simulink model "main1"  (Simulink 7.5)
settings: Solver=ode45  StartTime=0.0  StopTime=0.5  RelTol=1e-3
undefined symbols (not defined in the file or in its folder): D1, Delta, DiscIntNeverNeededParam, Hydride, Metal, Nickel
libraries: elec_lib x216, powerlib x83, fl_lib x9, powerlib_extras x8, simulink x3, nesl_utility x2, electricdrivelib x1
(part 1 of 2)
settings Model: Creator=quad  LastModifiedBy=quad

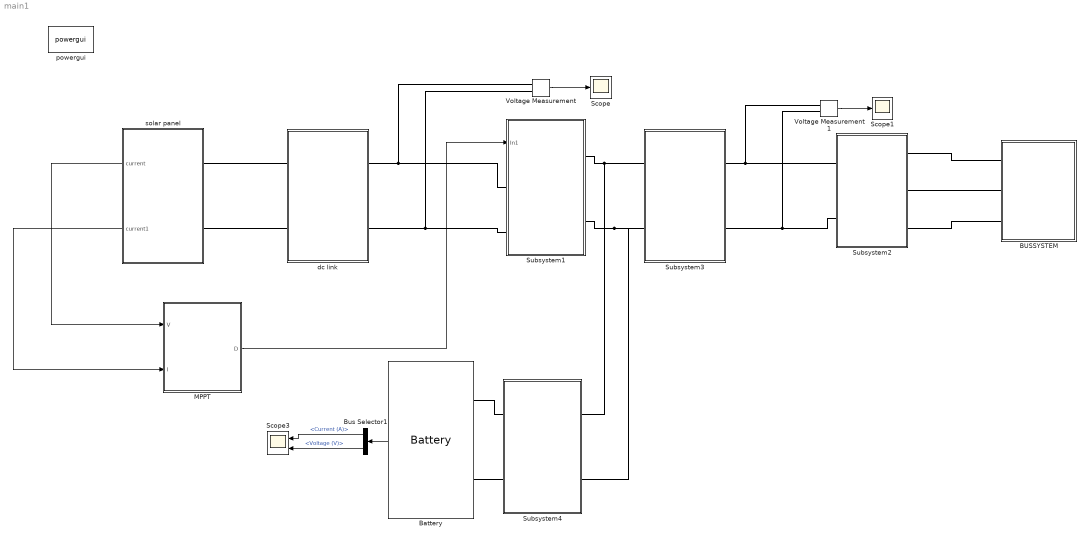
== system main1 ==
  BUSSYSTEM : Subsystem
  Battery : electricdrivelib/Extra Sources/Battery  DialogController=POWERSYS.PowerSysDialog  SystemSampleTime=-1  BatType=Nickel-Metal-Hydride  ShowDetailedParameters=off  NomV=220  NomQ=100  SOC=100  PresetModel=on  MaxQ=107.6923  FullV=259.1525  Dis_rate=20  R=0.022  Normal_OP=96.1538  expZone="[238.6441            20]"  Dis_Char=off  current=[6.5 13 32.5]  Units=Time  Batt_Tr=30
  Bus Selector1 : BusSelector  OutputSignals=Current (A),Voltage (V)
  MPPT : Subsystem
      mask Display: disp('MPPT')
  Scope : Scope
      settings: YMin=75  YMax=115  SaveName=ScopeData6
  Scope1 : Scope
      settings: YMin=0  YMax=1050
  Scope3 : Scope  NumInputPorts=2
      settings: YMin=-0.5~259.4  YMax=9~259.6  SaveName=ScopeData5
  Subsystem1 : Subsystem
      mask Display: disp('Converter')
  Subsystem2 : Subsystem
      mask Display: disp('Inverter')
  Subsystem3 : Subsystem
      mask Display: disp('DC Link')
  Subsystem4 : Subsystem
      mask Display: disp('Converter')
  Voltage Measurement : powerlib/Measurements/Voltage Measurement  DialogController=POWERSYS.PowerSysDialog  SystemSampleTime=-1  PhasorSimulation=off  OutputType=Complex  PSBequivalent=0
  Voltage Measurement1 : powerlib/Measurements/Voltage Measurement  DialogController=POWERSYS.PowerSysDialog  SystemSampleTime=-1  PhasorSimulation=off  OutputType=Complex  PSBequivalent=0
  dc link : Subsystem
      mask Display: disp('DC Link')
  powergui : powerlib/powergui  Priority=1  SystemSampleTime=-1  SimulationMode=Discrete  SampleTime=5e-6  frequency=60  SPID=off  DisableSnubberDevices=off  DisableRonSwitches=off  DisableVfSwitches=off  SwTol=0  Interpol=off  frequencyindice=50  echomessages=off  HookPort=off  DisplayEquations=off  FunctionMessages=off  EnableUseOfTLC=off  x0status=blocks  RestoreLinks=warning  ResistiveCurrentMeasurement=off  Ylog=off  Xlog=on  ShowGrid=off  save=off  variable=ZData  ZoomFFT=off  StartTime=0.0  cycles=1  DisplayStyle=1  FreqAxis=off  MaxFrequency=1000  frequencyindicesteady=1  display=off  methode=off
  solar panel : Subsystem
      mask Display: disp('Solar Panel')
  wires:
  Voltage Measurement/1 -> Scope/1
  Voltage Measurement1/1 -> Scope1/1
  Battery/1 -> Bus Selector1/1
  Bus Selector1/1 -> Scope3/1  "<Current (A)>"
  Bus Selector1/2 -> Scope3/2  "<Voltage (V)>"
  solar panel/1(current) -> MPPT/1(V)
  solar panel/2(current1) -> MPPT/2(I)
  MPPT/1(D) -> Subsystem1/1(In1)
  connections:
  Voltage Measurement/LConn1 -- dc link/RConn1 -- Subsystem1/LConn1
  Voltage Measurement/LConn2 -- dc link/RConn2 -- Subsystem1/LConn2
  Subsystem4/RConn1 -- Subsystem1/RConn1 -- Subsystem3/LConn1
  Subsystem4/RConn2 -- Subsystem1/RConn2 -- Subsystem3/LConn2
  Subsystem2/LConn1 -- Voltage Measurement1/LConn1 -- Subsystem3/RConn1
  Subsystem2/LConn2 -- Voltage Measurement1/LConn2 -- Subsystem3/RConn2
  Battery/LConn2 -- Subsystem4/LConn2
  solar panel/LConn2 -- dc link/LConn2
  solar panel/LConn1 -- dc link/LConn1
  Battery/LConn1 -- Subsystem4/LConn1
  Subsystem2/RConn1 -- BUSSYSTEM/LConn1
  Subsystem2/RConn2 -- BUSSYSTEM/LConn2
  Subsystem2/RConn3 -- BUSSYSTEM/LConn3

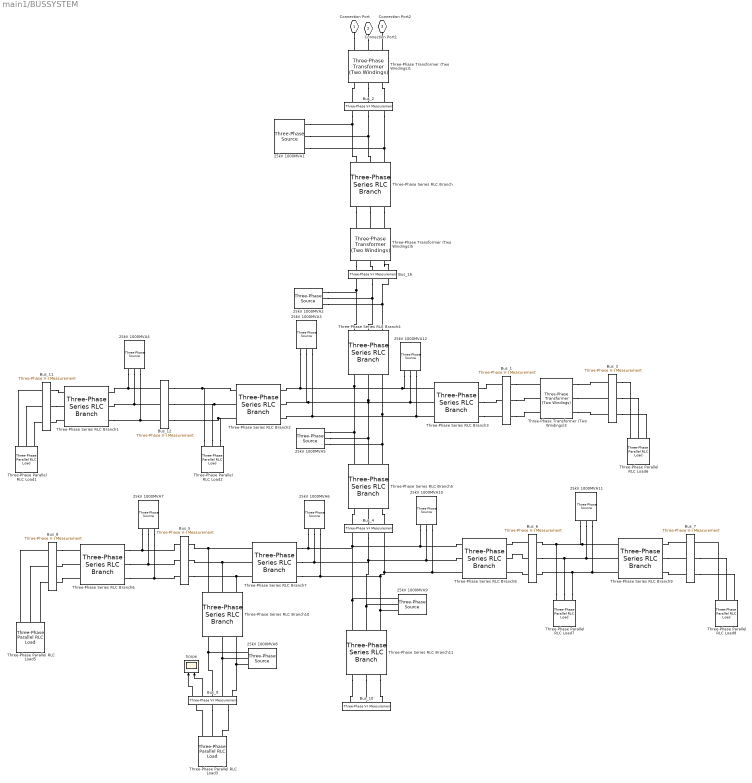
== system main1/BUSSYSTEM ==
  25kV 1000MVA{1..4,6..12} (11 alike) : powerlib/Electrical Sources/Three-Phase Source  DialogController=POWERSYS.PowerSysDialog  SystemSampleTime=-1  Voltage=10  PhaseAngle=0  Frequency=50  InternalConnection=Yg  SpecifyImpedance=on  Resistance=25^2/1000/10  Inductance=25^2/1000/377  ShortCircuitLevel=1000e6  BaseVoltage=25e3  XRratio=10
  25kV 1000MVA5 : powerlib/Electrical Sources/Three-Phase Source  DialogController=POWERSYS.PowerSysDialog  SystemSampleTime=-1  Voltage=25e3  PhaseAngle=0  Frequency=50  InternalConnection=Yg  SpecifyImpedance=on  Resistance=25^2/1000/10  Inductance=25^2/1000/377  ShortCircuitLevel=1000e6  BaseVoltage=25e3  XRratio=10
  Bus_1 : powerlib/Measurements/Three-Phase V-I Measurement  DialogController=POWERSYS.PowerSysDialog  SystemSampleTime=-1  VoltageMeasurement=phase-to-phase  SetLabelV=on  LabelV=Vabc_5  Vpu=off  VpuLL=off  CurrentMeasurement=yes  SetLabelI=on  LabelI=Iabc_5  Ipu=off  Pbase=100e6  Vbase=120e3  OutputType=Complex  PhasorSimulation=on  PSBequivalent=0
      link override Model/VI/Ia: GotoTag=LibraryTag_Ia
      link override Model/VI/Ib: GotoTag=LibraryTag_Ib
      link override Model/VI/Ic: GotoTag=LibraryTag_Ic
      link override Model/VI/Va: GotoTag=LibraryTag_Va
      link override Model/VI/Vb: GotoTag=LibraryTag_Vb
      link override Model/VI/Vc: GotoTag=LibraryTag_Vc
  Bus_10 : powerlib/Measurements/Three-Phase V-I Measurement  DialogController=POWERSYS.PowerSysDialog  SystemSampleTime=-1  VoltageMeasurement=phase-to-phase  SetLabelV=on  LabelV=Vabc_13  Vpu=off  VpuLL=off  CurrentMeasurement=yes  SetLabelI=on  LabelI=Iabc_13  Ipu=off  Pbase=100e6  Vbase=120e3  OutputType=Complex  PhasorSimulation=on  PSBequivalent=0
      link override Model/VI/Ia: GotoTag=LibraryTag_Ia
      link override Model/VI/Ib: GotoTag=LibraryTag_Ib
      link override Model/VI/Ic: GotoTag=LibraryTag_Ic
      link override Model/VI/Va: GotoTag=LibraryTag_Va
      link override Model/VI/Vb: GotoTag=LibraryTag_Vb
      link override Model/VI/Vc: GotoTag=LibraryTag_Vc
  Bus_11 : powerlib/Measurements/Three-Phase V-I Measurement  DialogController=POWERSYS.PowerSysDialog  SystemSampleTime=-1  VoltageMeasurement=phase-to-phase  SetLabelV=on  LabelV=Vabc_3  Vpu=off  VpuLL=off  CurrentMeasurement=yes  SetLabelI=on  LabelI=Iabc_3  Ipu=off  Pbase=100e6  Vbase=120e3  OutputType=Complex  PhasorSimulation=on  PSBequivalent=0
      link override Model/VI/Ia: GotoTag=LibraryTag_Ia
      link override Model/VI/Ib: GotoTag=LibraryTag_Ib
      link override Model/VI/Ic: GotoTag=LibraryTag_Ic
      link override Model/VI/Va: GotoTag=LibraryTag_Va
      link override Model/VI/Vb: GotoTag=LibraryTag_Vb
      link override Model/VI/Vc: GotoTag=LibraryTag_Vc
  Bus_12 : powerlib/Measurements/Three-Phase V-I Measurement  DialogController=POWERSYS.PowerSysDialog  SystemSampleTime=-1  VoltageMeasurement=phase-to-phase  SetLabelV=on  LabelV=Vabc_4  Vpu=off  VpuLL=off  CurrentMeasurement=yes  SetLabelI=on  LabelI=Iabc_4  Ipu=off  Pbase=100e6  Vbase=120e3  OutputType=Complex  PhasorSimulation=on  PSBequivalent=0
      link override Model/VI/Ia: GotoTag=LibraryTag_Ia
      link override Model/VI/Ib: GotoTag=LibraryTag_Ib
      link override Model/VI/Ic: GotoTag=LibraryTag_Ic
      link override Model/VI/Va: GotoTag=LibraryTag_Va
      link override Model/VI/Vb: GotoTag=LibraryTag_Vb
      link override Model/VI/Vc: GotoTag=LibraryTag_Vc
  Bus_16 : powerlib/Measurements/Three-Phase V-I Measurement  DialogController=POWERSYS.PowerSysDialog  SystemSampleTime=-1  VoltageMeasurement=phase-to-phase  SetLabelV=on  LabelV=Vabc_1  Vpu=off  VpuLL=off  CurrentMeasurement=yes  SetLabelI=on  LabelI=Iabc_1  Ipu=off  Pbase=100e6  Vbase=120e3  OutputType=Complex  PhasorSimulation=on  PSBequivalent=0
      link override Model/VI/Ia: GotoTag=LibraryTag_Ia
      link override Model/VI/Ib: GotoTag=LibraryTag_Ib
      link override Model/VI/Ic: GotoTag=LibraryTag_Ic
      link override Model/VI/Va: GotoTag=LibraryTag_Va
      link override Model/VI/Vb: GotoTag=LibraryTag_Vb
      link override Model/VI/Vc: GotoTag=LibraryTag_Vc
  Bus_2 : powerlib/Measurements/Three-Phase V-I Measurement  DialogController=POWERSYS.PowerSysDialog  SystemSampleTime=-1  VoltageMeasurement=phase-to-phase  SetLabelV=on  LabelV=Vabc_2  Vpu=off  VpuLL=off  CurrentMeasurement=yes  SetLabelI=on  LabelI=Iabc_2  Ipu=off  Pbase=100e6  Vbase=120e3  OutputType=Complex  PhasorSimulation=on  PSBequivalent=0
      link override Model/VI/Ia: GotoTag=LibraryTag_Ia
      link override Model/VI/Ib: GotoTag=LibraryTag_Ib
      link override Model/VI/Ic: GotoTag=LibraryTag_Ic
      link override Model/VI/Va: GotoTag=LibraryTag_Va
      link override Model/VI/Vb: GotoTag=LibraryTag_Vb
      link override Model/VI/Vc: GotoTag=LibraryTag_Vc
  Bus_3 : powerlib/Measurements/Three-Phase V-I Measurement  DialogController=POWERSYS.PowerSysDialog  SystemSampleTime=-1  VoltageMeasurement=phase-to-phase  SetLabelV=on  LabelV=Vabc_6  Vpu=off  VpuLL=off  CurrentMeasurement=yes  SetLabelI=on  LabelI=Iabc_6  Ipu=off  Pbase=100e6  Vbase=120e3  OutputType=Complex  PhasorSimulation=on  PSBequivalent=0
      link override Model/VI/Ia: GotoTag=LibraryTag_Ia
      link override Model/VI/Ib: GotoTag=LibraryTag_Ib
      link override Model/VI/Ic: GotoTag=LibraryTag_Ic
      link override Model/VI/Va: GotoTag=LibraryTag_Va
      link override Model/VI/Vb: GotoTag=LibraryTag_Vb
      link override Model/VI/Vc: GotoTag=LibraryTag_Vc
  Bus_4 : powerlib/Measurements/Three-Phase V-I Measurement  DialogController=POWERSYS.PowerSysDialog  SystemSampleTime=-1  VoltageMeasurement=phase-to-phase  SetLabelV=on  LabelV=Vabc_7  Vpu=off  VpuLL=off  CurrentMeasurement=yes  SetLabelI=on  LabelI=Iabc_7  Ipu=off  Pbase=100e6  Vbase=120e3  OutputType=Complex  PhasorSimulation=on  PSBequivalent=0
      link override Model/VI/Ia: GotoTag=LibraryTag_Ia
      link override Model/VI/Ib: GotoTag=LibraryTag_Ib
      link override Model/VI/Ic: GotoTag=LibraryTag_Ic
      link override Model/VI/Va: GotoTag=LibraryTag_Va
      link override Model/VI/Vb: GotoTag=LibraryTag_Vb
      link override Model/VI/Vc: GotoTag=LibraryTag_Vc
  Bus_5 : powerlib/Measurements/Three-Phase V-I Measurement  DialogController=POWERSYS.PowerSysDialog  SystemSampleTime=-1  VoltageMeasurement=phase-to-phase  SetLabelV=on  LabelV=Vabc_8  Vpu=off  VpuLL=off  CurrentMeasurement=yes  SetLabelI=on  LabelI=Iabc_8  Ipu=off  Pbase=100e6  Vbase=120e3  OutputType=Complex  PhasorSimulation=on  PSBequivalent=0
      link override Model/VI/Ia: GotoTag=LibraryTag_Ia
      link override Model/VI/Ib: GotoTag=LibraryTag_Ib
      link override Model/VI/Ic: GotoTag=LibraryTag_Ic
      link override Model/VI/Va: GotoTag=LibraryTag_Va
      link override Model/VI/Vb: GotoTag=LibraryTag_Vb
      link override Model/VI/Vc: GotoTag=LibraryTag_Vc
  Bus_6 : powerlib/Measurements/Three-Phase V-I Measurement  DialogController=POWERSYS.PowerSysDialog  SystemSampleTime=-1  VoltageMeasurement=phase-to-phase  SetLabelV=on  LabelV=Vabc_10  Vpu=off  VpuLL=off  CurrentMeasurement=yes  SetLabelI=on  LabelI=Iabc_10  Ipu=off  Pbase=100e6  Vbase=120e3  OutputType=Complex  PhasorSimulation=on  PSBequivalent=0
      link override Model/VI/Ia: GotoTag=LibraryTag_Ia
      link override Model/VI/Ib: GotoTag=LibraryTag_Ib
      link override Model/VI/Ic: GotoTag=LibraryTag_Ic
      link override Model/VI/Va: GotoTag=LibraryTag_Va
      link override Model/VI/Vb: GotoTag=LibraryTag_Vb
      link override Model/VI/Vc: GotoTag=LibraryTag_Vc
  Bus_7 : powerlib/Measurements/Three-Phase V-I Measurement  DialogController=POWERSYS.PowerSysDialog  SystemSampleTime=-1  VoltageMeasurement=phase-to-phase  SetLabelV=on  LabelV=Vabc_11  Vpu=off  VpuLL=off  CurrentMeasurement=yes  SetLabelI=on  LabelI=Iabc_11  Ipu=off  Pbase=100e6  Vbase=120e3  OutputType=Complex  PhasorSimulation=on  PSBequivalent=0
      link override Model/VI/Ia: GotoTag=LibraryTag_Ia
      link override Model/VI/Ib: GotoTag=LibraryTag_Ib
      link override Model/VI/Ic: GotoTag=LibraryTag_Ic
      link override Model/VI/Va: GotoTag=LibraryTag_Va
      link override Model/VI/Vb: GotoTag=LibraryTag_Vb
      link override Model/VI/Vc: GotoTag=LibraryTag_Vc
  Bus_8 : powerlib/Measurements/Three-Phase V-I Measurement  DialogController=POWERSYS.PowerSysDialog  SystemSampleTime=-1  VoltageMeasurement=phase-to-phase  SetLabelV=on  LabelV=Vabc_9  Vpu=off  VpuLL=off  CurrentMeasurement=yes  SetLabelI=on  LabelI=Iabc_9  Ipu=off  Pbase=100e6  Vbase=120e3  OutputType=Complex  PhasorSimulation=on  PSBequivalent=0
      link override Model/VI/Ia: GotoTag=LibraryTag_Ia
      link override Model/VI/Ib: GotoTag=LibraryTag_Ib
      link override Model/VI/Ic: GotoTag=LibraryTag_Ic
      link override Model/VI/Va: GotoTag=LibraryTag_Va
      link override Model/VI/Vb: GotoTag=LibraryTag_Vb
      link override Model/VI/Vc: GotoTag=LibraryTag_Vc
  Bus_9 : powerlib/Measurements/Three-Phase V-I Measurement  DialogController=POWERSYS.PowerSysDialog  SystemSampleTime=-1  VoltageMeasurement=phase-to-phase  SetLabelV=off  LabelV=Vabc_12  Vpu=off  VpuLL=off  CurrentMeasurement=yes  SetLabelI=off  LabelI=Iabc_12  Ipu=off  Pbase=100e6  Vbase=120e3  OutputType=Complex  PhasorSimulation=on  PSBequivalent=0
      link override Model/VI/Ia: GotoTag=LibraryTag_Ia
      link override Model/VI/Ib: GotoTag=LibraryTag_Ib
      link override Model/VI/Ic: GotoTag=LibraryTag_Ic
      link override Model/VI/Va: GotoTag=LibraryTag_Va
      link override Model/VI/Vb: GotoTag=LibraryTag_Vb
      link override Model/VI/Vc: GotoTag=LibraryTag_Vc
  Scope : Scope  NumInputPorts=2
      settings: YMin=-8~-0.4  YMax=14~0.45  SaveName=ScopeData4
  Three-Phase Parallel RLC Load{1..3,5..8} (7 alike) : powerlib/Elements/Three-Phase Parallel RLC Load  DialogController=POWERSYS.PowerSysDialog  PhysicalDomain=powersysdomain  SubClassName=unknown  LeftPortType=p1  RightPortType=p1  LConnTagsString=A|B|C  Configuration=Y (grounded)  NominalVoltage=415  NominalFrequency=50  ActivePower=10e3  InductivePower=0  CapacitivePower=0  Measurements=None
  Three-Phase Series RLC Branch{,1..11} (12 alike) : powerlib/Elements/Three-Phase Series RLC Branch  DialogController=POWERSYS.PowerSysDialog  PhysicalDomain=powersysdomain  SubClassName=unknown  LeftPortType=p1  RightPortType=p1  LConnTagsString=A|B|C  RConnTagsString=A|B|C  BranchType=RL  Resistance=10  Inductance=1e-3  Capacitance=1e-6  Measurements=None
  Three-Phase Transformer (Two Windings)1 : powerlib/Elements/Three-Phase Transformer (Two Windings)  DialogController=POWERSYS.PowerSysDialog  SystemSampleTime=-1  Winding1Connection=Delta (D1)  UNITS=pu  NominalPower=[ 1 , 50 ]  Winding1=[ 1.06 , 0.002 , 0.08 ]  Winding2Connection=Yg  Winding2=[100 , 0.002 , 0.08 ]  SetSaturation=off  Rm=500  Lm=500  Saturation=[ 0,0 ; 0.0024,1.2 ; 1.0,1.52 ]  Hysteresis=off  DataFile='hysteresis'  SetInitialFlux=off  InitialFluxes=[ 0.8 , -0.8 , 0.7 ]  Measurements=None  MoreParameters=off  BreakLoop=off  DataType=off  TransfoNumber=1
  Three-Phase Transformer (Two Windings)3 : powerlib/Elements/Three-Phase Transformer (Two Windings)  DialogController=POWERSYS.PowerSysDialog  SystemSampleTime=-1  Winding1Connection=Delta (D1)  UNITS=pu  NominalPower=[ 1 , 50 ]  Winding1=[ 1.06 , 0.002 , 0.08 ]  Winding2Connection=Yg  Winding2=[ 1.06 , 0.002 , 0.08 ]  SetSaturation=off  Rm=500  Lm=500  Saturation=[ 0,0 ; 0.0024,1.2 ; 1.0,1.52 ]  Hysteresis=off  DataFile='hysteresis'  SetInitialFlux=off  InitialFluxes=[ 0.8 , -0.8 , 0.7 ]  Measurements=None  MoreParameters=off  BreakLoop=off  DataType=off  TransfoNumber=1
  Three-Phase Transformer (Two Windings)5 : powerlib/Elements/Three-Phase Transformer (Two Windings)  DialogController=POWERSYS.PowerSysDialog  SystemSampleTime=-1  Winding1Connection=Delta (D1)  UNITS=pu  NominalPower=[ 1 , 50 ]  Winding1=[ 1.06 , 0.002 , 0.08 ]  Winding2Connection=Yg  Winding2=[1000 , 0.002 , 0.08 ]  SetSaturation=off  Rm=500  Lm=500  Saturation=[ 0,0 ; 0.0024,1.2 ; 1.0,1.52 ]  Hysteresis=off  DataFile='hysteresis'  SetInitialFlux=off  InitialFluxes=[ 0.8 , -0.8 , 0.7 ]  Measurements=None  MoreParameters=off  BreakLoop=off  DataType=off  TransfoNumber=1
  Connection Port : PMIOPort  Tag=PMCPort  Port=1  Side=Left
  Connection Port1 : PMIOPort  Tag=PMCPort  Port=2  Side=Left
  Connection Port2 : PMIOPort  Tag=PMCPort  Port=3  Side=Left
  wires:
  Bus_9/1 -> Scope/1
  Bus_9/2 -> Scope/2
  connections:
  Three-Phase Parallel RLC Load2/LConn3 -- Bus_12/RConn3 -- Three-Phase Series RLC Branch2/LConn3
  Three-Phase Parallel RLC Load2/LConn2 -- Bus_12/RConn2 -- Three-Phase Series RLC Branch2/LConn2
  Three-Phase Parallel RLC Load2/LConn1 -- Bus_12/RConn1 -- Three-Phase Series RLC Branch2/LConn1
  Three-Phase Series RLC Branch10/RConn2 -- Bus_5/RConn2 -- Three-Phase Series RLC Branch7/LConn2
  Three-Phase Series RLC Branch10/RConn3 -- Bus_5/RConn3 -- Three-Phase Series RLC Branch7/LConn3
  Three-Phase Series RLC Branch10/RConn1 -- Bus_5/RConn1 -- Three-Phase Series RLC Branch7/LConn1
  25kV 1000MVA12/RConn1 -- Three-Phase Series RLC Branch4/RConn1 -- Three-Phase Series RLC Branch2/RConn1 -- 25kV 1000MVA3/RConn1 -- Three-Phase Series RLC Branch5/LConn1 -- 25kV 1000MVA5/RConn1 -- Three-Phase Series RLC Branch3/LConn1
  25kV 1000MVA12/RConn2 -- Three-Phase Series RLC Branch2/RConn2 -- 25kV 1000MVA3/RConn2 -- Three-Phase Series RLC Branch5/LConn2 -- 25kV 1000MVA5/RConn2 -- Three-Phase Series RLC Branch4/RConn2 -- Three-Phase Series RLC Branch3/LConn2
  25kV 1000MVA12/RConn3 -- Three-Phase Series RLC Branch4/RConn3 -- Three-Phase Series RLC Branch2/RConn3 -- 25kV 1000MVA3/RConn3 -- Three-Phase Series RLC Branch5/LConn3 -- 25kV 1000MVA5/RConn3 -- Three-Phase Series RLC Branch3/LConn3
  25kV 1000MVA10/RConn1 -- Bus_4/LConn1 -- Three-Phase Series RLC Branch7/RConn1 -- 25kV 1000MVA6/RConn1 -- Three-Phase Series RLC Branch11/LConn1 -- 25kV 1000MVA9/RConn1 -- Three-Phase Series RLC Branch8/LConn1
  25kV 1000MVA10/RConn2 -- Bus_4/LConn2 -- Three-Phase Series RLC Branch7/RConn2 -- 25kV 1000MVA6/RConn2 -- Three-Phase Series RLC Branch11/LConn2 -- 25kV 1000MVA9/RConn2 -- Three-Phase Series RLC Branch8/LConn2
  25kV 1000MVA10/RConn3 -- Bus_4/LConn3 -- Three-Phase Series RLC Branch7/RConn3 -- 25kV 1000MVA6/RConn3 -- Three-Phase Series RLC Branch11/LConn3 -- 25kV 1000MVA9/RConn3 -- Three-Phase Series RLC Branch8/LConn3
  25kV 1000MVA4/RConn3 -- Three-Phase Series RLC Branch1/RConn3 -- Bus_12/LConn3
  25kV 1000MVA1/RConn3 -- Bus_2/LConn3 -- Three-Phase Series RLC Branch/LConn3
  25kV 1000MVA8/RConn3 -- Bus_9/RConn3 -- Three-Phase Series RLC Branch10/LConn3
  Three-Phase Parallel RLC Load7/LConn1 -- Bus_6/RConn1 -- Three-Phase Series RLC Branch9/LConn1 -- 25kV 1000MVA11/RConn1
  25kV 1000MVA4/RConn1 -- Three-Phase Series RLC Branch1/RConn1 -- Bus_12/LConn1
  25kV 1000MVA2/RConn2 -- Bus_16/LConn2 -- Three-Phase Series RLC Branch4/LConn2
  25kV 1000MVA2/RConn3 -- Bus_16/LConn3 -- Three-Phase Series RLC Branch4/LConn3
  25kV 1000MVA8/RConn1 -- Bus_9/RConn1 -- Three-Phase Series RLC Branch10/LConn1
  25kV 1000MVA2/RConn1 -- Three-Phase Series RLC Branch4/LConn1 -- Bus_16/LConn1
  25kV 1000MVA4/RConn2 -- Three-Phase Series RLC Branch1/RConn2 -- Bus_12/LConn2
  25kV 1000MVA7/RConn1 -- Three-Phase Series RLC Branch6/RConn1 -- Bus_5/LConn1
  Three-Phase Parallel RLC Load7/LConn2 -- Bus_6/RConn2 -- Three-Phase Series RLC Branch9/LConn2 -- 25kV 1000MVA11/RConn2
  25kV 1000MVA8/RConn2 -- Bus_9/RConn2 -- Three-Phase Series RLC Branch10/LConn2
  25kV 1000MVA1/RConn2 -- Bus_2/LConn2 -- Three-Phase Series RLC Branch/LConn2
  25kV 1000MVA1/RConn1 -- Bus_2/LConn1 -- Three-Phase Series RLC Branch/LConn1
  25kV 1000MVA7/RConn2 -- Three-Phase Series RLC Branch6/RConn2 -- Bus_5/LConn2
  25kV 1000MVA7/RConn3 -- Three-Phase Series RLC Branch6/RConn3 -- Bus_5/LConn3
  Three-Phase Parallel RLC Load7/LConn3 -- Bus_6/RConn3 -- Three-Phase Series RLC Branch9/LConn3 -- 25kV 1000MVA11/RConn3
  Three-Phase Series RLC Branch/RConn1 -- Three-Phase Transformer (Two Windings)5/LConn1
  Bus_7/RConn2 -- Three-Phase Parallel RLC Load8/LConn2
  Three-Phase Parallel RLC Load1/LConn2 -- Bus_11/LConn2
  Three-Phase Series RLC Branch5/RConn3 -- Bus_4/RConn3
  Three-Phase Transformer (Two Windings)3/LConn3 -- Bus_3/LConn3
  Bus_6/LConn2 -- Three-Phase Series RLC Branch8/RConn2
  Bus_1/RConn2 -- Three-Phase Transformer (Two Windings)3/RConn2
  Bus_11/RConn3 -- Three-Phase Series RLC Branch1/LConn3
  Bus_6/LConn3 -- Three-Phase Series RLC Branch8/RConn3
  Bus_8/RConn2 -- Three-Phase Series RLC Branch6/LConn2
  Three-Phase Parallel RLC Load5/LConn2 -- Bus_8/LConn2
  Three-Phase Series RLC Branch/RConn3 -- Three-Phase Transformer (Two Windings)5/LConn3
  Bus_7/RConn3 -- Three-Phase Parallel RLC Load8/LConn3
  Bus_3/RConn1 -- Three-Phase Parallel RLC Load6/LConn1
  Three-Phase Parallel RLC Load8/LConn1 -- Bus_7/RConn1
  Three-Phase Parallel RLC Load5/LConn1 -- Bus_8/LConn1
  Three-Phase Series RLC Branch11/RConn1 -- Bus_10/RConn1
  Three-Phase Transformer (Two Windings)1/RConn3 -- Bus_2/RConn3
  Three-Phase Series RLC Branch9/RConn2 -- Bus_7/LConn2
  Bus_11/RConn2 -- Three-Phase Series RLC Branch1/LConn2
  Three-Phase Series RLC Branch3/RConn3 -- Bus_1/LConn3
  Bus_9/LConn2 -- Three-Phase Parallel RLC Load3/LConn2
  Three-Phase Transformer (Two Windings)3/LConn1 -- Bus_3/LConn1
  Three-Phase Series RLC Branch3/RConn1 -- Bus_1/LConn1
  Three-Phase Parallel RLC Load5/LConn3 -- Bus_8/LConn3
  Three-Phase Parallel RLC Load1/LConn3 -- Bus_11/LConn3
  Three-Phase Transformer (Two Windings)5/RConn2 -- Bus_16/RConn2
  Three-Phase Series RLC Branch3/RConn2 -- Bus_1/LConn2
  Three-Phase Series RLC Branch9/RConn3 -- Bus_7/LConn3
  Bus_9/LConn3 -- Three-Phase Parallel RLC Load3/LConn3
  Bus_6/LConn1 -- Three-Phase Series RLC Branch8/RConn1
  Bus_1/RConn3 -- Three-Phase Transformer (Two Windings)3/RConn3
  Bus_4/RConn2 -- Three-Phase Series RLC Branch5/RConn2
  Bus_3/RConn3 -- Three-Phase Parallel RLC Load6/LConn3
  Bus_8/RConn3 -- Three-Phase Series RLC Branch6/LConn3
  Three-Phase Series RLC Branch11/RConn2 -- Bus_10/RConn2
  Bus_1/RConn1 -- Three-Phase Transformer (Two Windings)3/RConn1
  Three-Phase Series RLC Branch11/RConn3 -- Bus_10/RConn3
  Three-Phase Transformer (Two Windings)3/LConn2 -- Bus_3/LConn2
  Three-Phase Transformer (Two Windings)1/RConn2 -- Bus_2/RConn2
  Bus_3/RConn2 -- Three-Phase Parallel RLC Load6/LConn2
  Three-Phase Transformer (Two Windings)5/RConn1 -- Bus_16/RConn1
  Three-Phase Series RLC Branch9/RConn1 -- Bus_7/LConn1
  Three-Phase Parallel RLC Load3/LConn1 -- Bus_9/LConn1
  Bus_11/RConn1 -- Three-Phase Series RLC Branch1/LConn1
  Three-Phase Parallel RLC Load1/LConn1 -- Bus_11/LConn1
  Bus_4/RConn1 -- Three-Phase Series RLC Branch5/RConn1
  Three-Phase Transformer (Two Windings)1/RConn1 -- Bus_2/RConn1
  Three-Phase Series RLC Branch/RConn2 -- Three-Phase Transformer (Two Windings)5/LConn2
  Three-Phase Transformer (Two Windings)5/RConn3 -- Bus_16/RConn3
  Connection Port1/RConn1 -- Three-Phase Transformer (Two Windings)1/LConn2
  Bus_8/RConn1 -- Three-Phase Series RLC Branch6/LConn1
  Connection Port/RConn1 -- Three-Phase Transformer (Two Windings)1/LConn1
  Connection Port2/RConn1 -- Three-Phase Transformer (Two Windings)1/LConn3

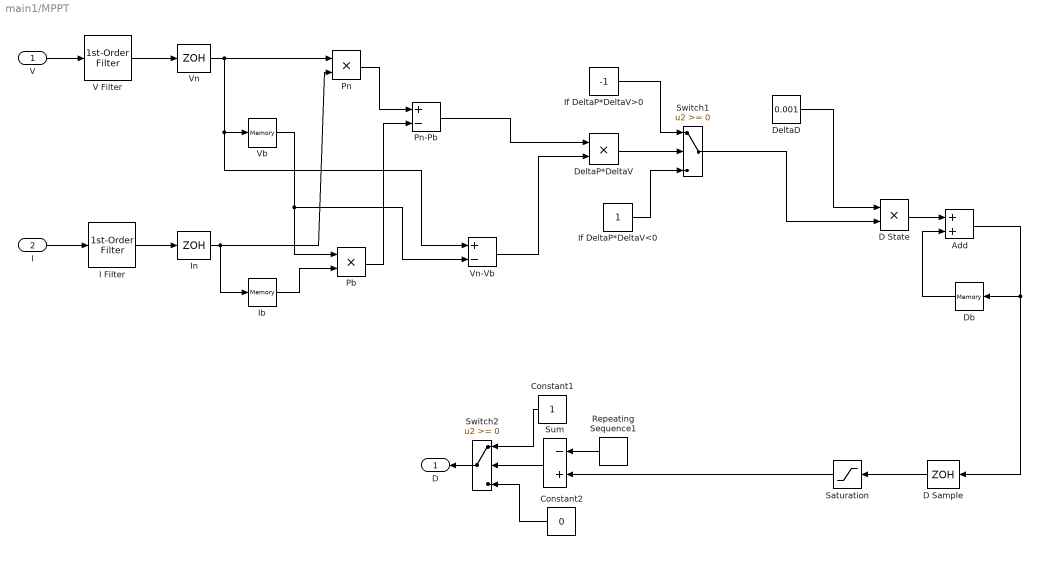
== system main1/MPPT ==
  V : Inport
  I : Inport  Port=2
  Add : Sum
  Constant1 : Constant  SampleTime=-1
  Constant2 : Constant  Value=0  SampleTime=-1
  D Sample : ZeroOrderHold  SampleTime=1e-4
  D State : Product  RndMeth=Zero
  Db : Memory  InheritSampleTime=on  LinearizeAsDelay=on
  DeltaD : Constant  Value=0.001
  DeltaP*DeltaV : Product  RndMeth=Zero
  I Filter : powerlib_extras/Control  Blocks/1st-Order  Filter  DialogController=POWERSYS.PowerSysDialog  SystemSampleTime=-1  FilterType=Lowpass  Tc=1e-3  Initialize=off  Vac_Init=[0.8 -25 60]  Vdc_Init=-0.4  PlotResponse=off  param1=[1 500 1]
  Ib : Memory  InheritSampleTime=on  LinearizeAsDelay=on
  If DeltaP*DeltaV<0 : Constant
  If DeltaP*DeltaV>0 : Constant  Value=-1
  In : ZeroOrderHold  SampleTime=1e-4
  Pb : Product  RndMeth=Zero
  Pn : Product  RndMeth=Zero
  Pn-Pb : Sum  Inputs=+-
  Repeating Sequence1 : simulink/Sources/Repeating Sequence  SystemSampleTime=-1  rep_seq_t=[0 4e-3 4e-3]  rep_seq_y=[0 1 0]
  Saturation : Saturate  UpperLimit=0.8  LowerLimit=0
  Sum : Sum  Inputs=-+  SaturateOnIntegerOverflow=on
  Switch1 : Switch
  Switch2 : Switch
  V Filter : powerlib_extras/Control  Blocks/1st-Order  Filter  DialogController=POWERSYS.PowerSysDialog  SystemSampleTime=-1  FilterType=Lowpass  Tc=1e-3  Initialize=off  Vac_Init=[0.8 -25 60]  Vdc_Init=-0.4  PlotResponse=off  param1=[1 500 1]
  Vb : Memory  InheritSampleTime=on  LinearizeAsDelay=on
  Vn : ZeroOrderHold  SampleTime=1e-4
  Vn-Vb : Sum  Inputs=+-
  D : Outport
  wires:
  V/1 -> V Filter/1
  I/1 -> I Filter/1
  V Filter/1 -> Vn/1
  I Filter/1 -> In/1
  In/1 -> Ib/1, Pn/2
  Vn/1 -> Pn/1, Vb/1, Vn-Vb/1
  Ib/1 -> Pb/2
  Vb/1 -> Pb/1, Vn-Vb/2
  Pn/1 -> Pn-Pb/1
  Pb/1 -> Pn-Pb/2
  D State/1 -> Add/1
  Constant2/1 -> Switch2/3
  Constant1/1 -> Switch2/1
  Sum/1 -> Switch2/2
  Repeating Sequence1/1 -> Sum/1
  Add/1 -> Db/1, D Sample/1
  Switch2/1 -> D/1
  Db/1 -> Add/2
  D Sample/1 -> Saturation/1
  Pn-Pb/1 -> DeltaP*DeltaV/1
  Vn-Vb/1 -> DeltaP*DeltaV/2
  DeltaP*DeltaV/1 -> Switch1/2
  If DeltaP*DeltaV>0/1 -> Switch1/1
  If DeltaP*DeltaV<0/1 -> Switch1/3
  Switch1/1 -> D State/2
  DeltaD/1 -> D State/1
  Saturation/1 -> Sum/2

== system main1/Subsystem1 ==
  In1 : Inport  OutDataType=fixdt(1, 16)  OutScaling=2^0
  "  " : powerlib/Measurements/Voltage Measurement  DialogController=POWERSYS.PowerSysDialog  SystemSampleTime=-1  PhasorSimulation=off  OutputType=Complex  PSBequivalent=0
  "    " : powerlib/Elements/Series RLC Branch  DialogController=POWERSYS.PowerSysDialog  PhysicalDomain=powersysdomain  SubClassName=unknown  LeftPortType=p1  RightPortType=p1  LConnTagsString=__new0  RConnTagsString=__new0  BranchType=RC  Resistance=1  Inductance=69e-3  SetiL0=off  InitialCurrent=0  Capacitance=9.6e-7  Setx0=off  InitialVoltage=0  Measurements=None
  " Measurement" : powerlib/Measurements/Voltage Measurement  DialogController=POWERSYS.PowerSysDialog  SystemSampleTime=-1  PhasorSimulation=off  OutputType=Complex  PSBequivalent=0
  " Measurement1" : powerlib/Measurements/Current Measurement  DialogController=POWERSYS.PowerSysDialog  SystemSampleTime=-1  PhasorSimulation=off  OutputType=Complex  PSBequivalent=0
  Diode : powerlib/Power Electronics/Diode  DialogController=POWERSYS.PowerSysDialog  SystemSampleTime=-1  Ron=0.001  Lon=0  Vf=0.8  IC=0  UseSnubber=off  Rs=500  Cs=250e-9  Measurements=on
  Mosfet : powerlib/Power Electronics/Mosfet  DialogController=POWERSYS.PowerSysDialog  SystemSampleTime=-1  Ron=0.1  Lon=0  Rd=0.01  Vfd=0  IC=0  Rs=1e5  Cs=inf  Measurements=on
  Scope : Scope  NumInputPorts=2
      settings: TimeRange=0.1  YMin=75~0  YMax=115~1050
  Series RLC Branch : powerlib/Elements/Series RLC Branch  DialogController=POWERSYS.PowerSysDialog  PhysicalDomain=powersysdomain  SubClassName=unknown  LeftPortType=p1  RightPortType=p1  LConnTagsString=__new0  RConnTagsString=__new0  BranchType=RL  Resistance=0  Inductance=2.332e-3  SetiL0=off  InitialCurrent=0  Capacitance=1e-6  Setx0=off  InitialVoltage=0  Measurements=None
  + : PMIOPort  Port=1  Side=Left
  _ : PMIOPort  Port=2  Side=Left
  ++ : PMIOPort  Port=3  Side=Right
  __ : PMIOPort  Port=4  Side=Right
  wires:
  " Measurement"/1 -> Scope/2
  "  "/1 -> Scope/1
  In1/1 -> Mosfet/1
  connections:
  Mosfet/LConn1 -- Series RLC Branch/RConn1 -- Diode/LConn1
  " Measurement"/LConn2 -- __/RConn1 -- "    "/RConn1 -- "  "/LConn2 -- _/RConn1 -- Mosfet/RConn1
  " Measurement1"/RConn1 -- " Measurement"/LConn1 -- ++/RConn1
  "    "/LConn1 -- " Measurement1"/LConn1 -- Diode/RConn1
  +/RConn1 -- Series RLC Branch/LConn1 -- "  "/LConn1

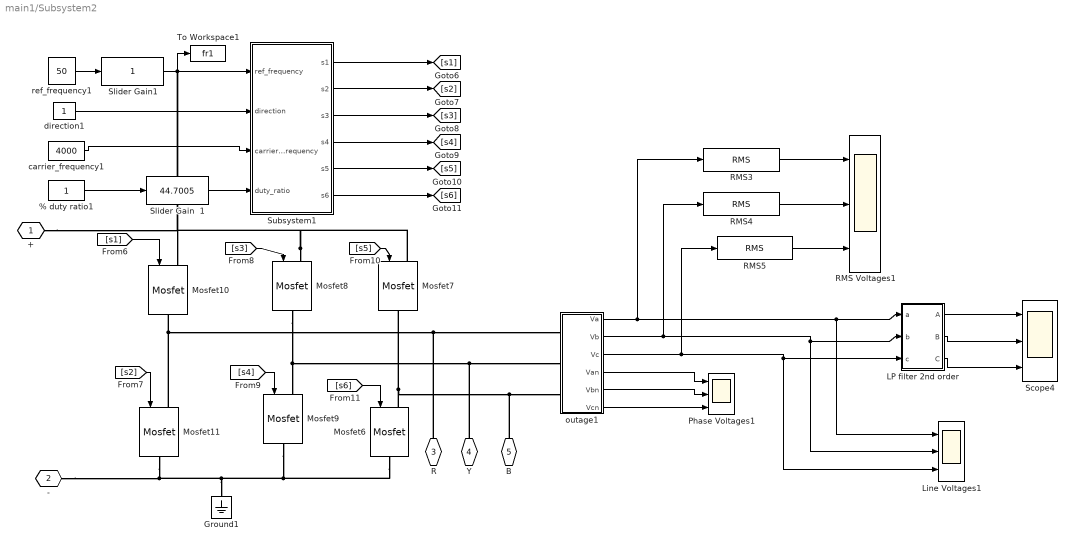
== system main1/Subsystem2 ==
  % duty ratio1 : Constant  OutDataType=fixdt(1, 16)  OutScaling=2^0
  Ground1 : powerlib/Elements/Ground  DialogController=POWERSYS.PowerSysDialog  PhysicalDomain=powersysdomain  SubClassName=unknown  LeftPortType=p1  RightPortType=p1  LConnTagsString=a
  LP filter 2nd order : Subsystem  mask{cutoff_frequency=100, damping_factor=0.707}
      mask prompts: cutoff_frequency "Cut off frequency"; damping_factor "Damping Factor"
  Line Voltages1 : Scope  NumInputPorts=3
      settings: TimeRange=0.1  YMin=-1250~-1250~-100  YMax=1250~1250~1100  SaveName=Line_voltages1  MaxDataPoints=50000  SampleInput=on  SampleTime=5e-6
  Mosfet{6..11} (6 alike) : powerlib/Power Electronics/Mosfet  DialogController=POWERSYS.PowerSysDialog  SystemSampleTime=-1  Ron=0.1  Lon=0  Rd=0.01  Vfd=0  IC=0  Rs=1e5  Cs=inf  Measurements=off
  Phase Voltages1 : Scope  NumInputPorts=3
      settings: TimeRange=0.1  YMin=-300~-300~-300  YMax=300~300~300  SaveName=Neutral_voltages2  MaxDataPoints=50000  SampleInput=on  SampleTime=5e-6
  RMS Voltages1 : Scope  NumInputPorts=3
      settings: TimeRange=0.1  YMin=438.25~396.75~418.75  YMax=440.75~399.5~421.5  SaveName=Neutral_voltages3  MaxDataPoints=50000  SampleInput=on  SampleTime=5e-6
  RMS3 : powerlib_extras/Measurements/RMS  DialogController=POWERSYS.PowerSysDialog  SystemSampleTime=-1  f1=60
  RMS4 : powerlib_extras/Measurements/RMS  DialogController=POWERSYS.PowerSysDialog  SystemSampleTime=-1  f1=60
  RMS5 : powerlib_extras/Measurements/RMS  DialogController=POWERSYS.PowerSysDialog  SystemSampleTime=-1  f1=60
  Scope4 : Scope  NumInputPorts=3
      settings: TimeRange=0.1  YMin=-1.45~-5.92~6.2  YMax=-0.5~-5.75~7.3  SaveName=Filtered_voltages  MaxDataPoints=5000000  SampleInput=on  SampleTime=5e-6
  Slider Gain  1 : simulink/Math Operations/Slider Gain  SystemSampleTime=-1  low=0  gain=44.7005  high=100
  Slider Gain1 : simulink/Math Operations/Slider Gain  SystemSampleTime=-1  low=0  gain=1  high=4
  Subsystem1 : Subsystem
  To Workspace1 : ToWorkspace  VariableName=fr1  SampleTime=-1  SaveFormat=Structure
  carrier_frequency1 : Constant  Value=4000  OutDataType=fixdt(1, 16)  OutScaling=2^0
  direction1 : Constant  OutDataType=fixdt(1, 16)  OutScaling=2^0
  outage1 : Subsystem
  ref_frequency1 : Constant  Value=50  OutDataType=fixdt(1, 16)  OutScaling=2^0
  + : PMIOPort  Tag=PMCPort  Port=1  Side=Left
  - : PMIOPort  Tag=PMCPort  Port=2  Side=Left
  R : PMIOPort  Tag=PMCPort  Port=3  Side=Right
  Y : PMIOPort  Tag=PMCPort  Port=4  Side=Right
  B : PMIOPort  Tag=PMCPort  Port=5  Side=Right
  wires:
  ref_frequency1/1 -> Slider Gain1/1
  direction1/1 -> Subsystem1/2(direction)
  [s1] -> Mosfet10/1
  [s2] -> Mosfet11/1
  [s3] -> Mosfet8/1
  [s4] -> Mosfet9/1
  [s5] -> Mosfet7/1
  [s6] -> Mosfet6/1
  outage1/4(Van) -> Phase Voltages1/1
  outage1/5(Vbn) -> Phase Voltages1/2
  outage1/6(Vcn) -> Phase Voltages1/3
  Subsystem1/1(s1) -> [s1]
  Subsystem1/2(s2) -> [s2]
  Subsystem1/3(s3) -> [s3]
  Subsystem1/4(s4) -> [s4]
  Subsystem1/5(s5) -> [s5]
  Subsystem1/6(s6) -> [s6]
  Slider Gain1/1 -> Subsystem1/1(ref_frequency), To Workspace1/1
  outage1/1(Va) -> RMS3/1, LP filter 2nd order/1(a), Line Voltages1/1
  outage1/2(Vb) -> RMS4/1, LP filter 2nd order/2(b), Line Voltages1/2
  outage1/3(Vc) -> RMS5/1, LP filter 2nd order/3(c), Line Voltages1/3
  carrier_frequency1/1 -> Subsystem1/3(carrier_frequency)
  % duty ratio1/1 -> Slider Gain  1/1
  Slider Gain  1/1 -> Subsystem1/4(duty_ratio)
  RMS3/1 -> RMS Voltages1/1
  RMS4/1 -> RMS Voltages1/2
  RMS5/1 -> RMS Voltages1/3
  LP filter 2nd order/2(B) -> Scope4/2
  LP filter 2nd order/1(A) -> Scope4/1
  LP filter 2nd order/3(C) -> Scope4/3
  connections:
  Mosfet8/LConn1 -- Mosfet7/LConn1 -- +/RConn1 -- Mosfet10/LConn1
  Mosfet11/LConn1 -- outage1/LConn1 -- R/RConn1 -- Mosfet10/RConn1
  Mosfet7/RConn1 -- outage1/LConn3 -- B/RConn1 -- Mosfet6/LConn1
  Ground1/LConn1 -- Mosfet6/RConn1 -- Mosfet9/RConn1 -- -/RConn1 -- Mosfet11/RConn1
  Mosfet8/RConn1 -- outage1/LConn2 -- Y/RConn1 -- Mosfet9/LConn1

== system main1/Subsystem3 ==
  Series RLC Branch : powerlib/Elements/Series RLC Branch  DialogController=POWERSYS.PowerSysDialog  PhysicalDomain=powersysdomain  SubClassName=unknown  LeftPortType=p1  RightPortType=p1  LConnTagsString=__new0  RConnTagsString=__new0  BranchType=C  Resistance=1  Inductance=1e-3  SetiL0=off  InitialCurrent=0  Capacitance=0.1e-6  Setx0=off  InitialVoltage=0  Measurements=None
  + : PMIOPort  Tag=PMCPort  Port=1  Side=Left
  _ : PMIOPort  Tag=PMCPort  Port=2  Side=Left
  ++ : PMIOPort  Tag=PMCPort  Port=3  Side=Right
  __ : PMIOPort  Tag=PMCPort  Port=4  Side=Right
  connections:
  __/RConn1 -- Series RLC Branch/RConn1 -- _/RConn1
  ++/RConn1 -- Series RLC Branch/LConn1 -- +/RConn1

== system main1/Subsystem4 ==
  "  " : powerlib/Measurements/Voltage Measurement  DialogController=POWERSYS.PowerSysDialog  SystemSampleTime=-1  PhasorSimulation=off  OutputType=Complex  PSBequivalent=0
  "    " : powerlib/Elements/Series RLC Branch  DialogController=POWERSYS.PowerSysDialog  PhysicalDomain=powersysdomain  SubClassName=unknown  LeftPortType=p1  RightPortType=p1  LConnTagsString=__new0  RConnTagsString=__new0  BranchType=RC  Resistance=0  Inductance=69e-3  SetiL0=off  InitialCurrent=0  Capacitance=9.6e-7  Setx0=off  InitialVoltage=0  Measurements=None
  " Measurement" : powerlib/Measurements/Voltage Measurement  DialogController=POWERSYS.PowerSysDialog  SystemSampleTime=-1  PhasorSimulation=off  OutputType=Complex  PSBequivalent=0
  " Measurement1" : powerlib/Measurements/Current Measurement  DialogController=POWERSYS.PowerSysDialog  SystemSampleTime=-1  PhasorSimulation=off  OutputType=Complex  PSBequivalent=0
  Diode : powerlib/Power Electronics/Diode  DialogController=POWERSYS.PowerSysDialog  SystemSampleTime=-1  Ron=0.001  Lon=0  Vf=0.8  IC=0  UseSnubber=off  Rs=500  Cs=250e-9  Measurements=on
  Mosfet : powerlib/Power Electronics/Mosfet  DialogController=POWERSYS.PowerSysDialog  SystemSampleTime=-1  Ron=0.1  Lon=0  Rd=0.01  Vfd=0  IC=0  Rs=1e5  Cs=inf  Measurements=on
  Pulse Generator : DiscretePulseGenerator  PulseType=Time based  Amplitude=1  Period=1/100000  PulseWidth=50  PhaseDelay=0  SampleTime=1
  Scope : Scope  NumInputPorts=2
      settings: TimeRange=0.1  YMin=259.4~0  YMax=259.6~1050
  Series RLC Branch : powerlib/Elements/Series RLC Branch  DialogController=POWERSYS.PowerSysDialog  PhysicalDomain=powersysdomain  SubClassName=unknown  LeftPortType=p1  RightPortType=p1  LConnTagsString=__new0  RConnTagsString=__new0  BranchType=RL  Resistance=0  Inductance=2.332e-3  SetiL0=off  InitialCurrent=0  Capacitance=1e-6  Setx0=off  InitialVoltage=0  Measurements=None
  + : PMIOPort  Port=1  Side=Left
  _ : PMIOPort  Port=2  Side=Left
  ++ : PMIOPort  Port=3  Side=Right
  __ : PMIOPort  Port=4  Side=Right
  wires:
  Pulse Generator/1 -> Mosfet/1
  "  "/1 -> Scope/1
  " Measurement"/1 -> Scope/2
  connections:
  "  "/LConn1 -- Series RLC Branch/LConn1 -- +/RConn1
  Diode/RConn1 -- " Measurement1"/LConn1 -- "    "/LConn1
  ++/RConn1 -- " Measurement"/LConn1 -- " Measurement1"/RConn1
  Mosfet/RConn1 -- _/RConn1 -- "  "/LConn2 -- "    "/RConn1 -- __/RConn1 -- " Measurement"/LConn2
  Diode/LConn1 -- Series RLC Branch/RConn1 -- Mosfet/LConn1

== system main1/dc link ==
  Series RLC Branch : powerlib/Elements/Series RLC Branch  DialogController=POWERSYS.PowerSysDialog  PhysicalDomain=powersysdomain  SubClassName=unknown  LeftPortType=p1  RightPortType=p1  LConnTagsString=__new0  RConnTagsString=__new0  BranchType=C  Resistance=1  Inductance=1e-3  SetiL0=off  InitialCurrent=0  Capacitance=0.1e-6  Setx0=off  InitialVoltage=0  Measurements=None
  + : PMIOPort  Tag=PMCPort  Port=1  Side=Left
  _ : PMIOPort  Tag=PMCPort  Port=2  Side=Left
  ++ : PMIOPort  Tag=PMCPort  Port=3  Side=Right
  __ : PMIOPort  Tag=PMCPort  Port=4  Side=Right
  connections:
  +/RConn1 -- Series RLC Branch/LConn1 -- ++/RConn1
  _/RConn1 -- Series RLC Branch/RConn1 -- __/RConn1

== system main1/solar panel ==
  " R " : powerlib/Elements/Series RLC Branch  DialogController=POWERSYS.PowerSysDialog  PhysicalDomain=powersysdomain  SubClassName=unknown  LeftPortType=p1  RightPortType=p1  LConnTagsString=__new0  RConnTagsString=__new0  BranchType=R  Resistance=10  Inductance=1e-3  SetiL0=off  InitialCurrent=0  Capacitance=1e-6  Setx0=off  InitialVoltage=0  Measurements=None
  Controlled  Current  Source : powerlib/Electrical Sources/Controlled Current Source  DialogController=POWERSYS.PowerSysDialog  SystemSampleTime=-1  Initialize=on  Source_Type=AC  Amplitude=0  Phase=0  Frequency=0  Measurements=None
  Current  Sensor : fl_lib/Electrical/Electrical Sensors/Current Sensor  DialogController=NetworkEngine.DynNeDlgSource  SystemSampleTime=-1  i1_Log=off  v1_Log=off  LocalVarNames=|i1|v1  LocalVarDescs=|i1|v1  LocalVarLogging=[0 0]
  Current  Measurement : powerlib/Measurements/Current Measurement  DialogController=POWERSYS.PowerSysDialog  SystemSampleTime=-1  PhasorSimulation=off  OutputType=Complex  PSBequivalent=0
  Electrical Reference : fl_lib/Electrical/Electrical Elements/Electrical Reference  DialogController=NetworkEngine.DynNeDlgSource  SystemSampleTime=-1  i_Log=off  LocalVarNames=|i  LocalVarDescs=|i  LocalVarLogging=0
  PS-Simulink Converter : nesl_utility/PS-Simulink Converter  DialogController=NetworkEngine.DynNeUtilDlgSource  SystemSampleTime=-1  PhysicalDomain=network_engine_domain  LeftPortType=input  RightPortType=output  SubClassName=ps_output  Unit=1  AffineConversion=off
  PV Pannel : Subsystem
  PV Pannel1 : Subsystem
  PV Pannel2 : Subsystem
  PV Pannel3 : Subsystem
  PV Pannel4 : Subsystem
  PV Pannel5 : Subsystem
  Product : Product  OutDataType=fixdt(1, 16)  OutScaling=2^0  RndMeth=Zero
  Scope1 : Scope  NumInputPorts=2
      settings: YMin=10.4699~75  YMax=10.4699~115  SaveName=ScopeData2
  Scope2 : Scope
      settings: YMin=0  YMax=1100  SaveName=ScopeData3
  Solver Configuration : nesl_utility/Solver Configuration  DialogController=NetworkEngine.DynNeUtilDlgSource  SystemSampleTime=-1  PhysicalDomain=network_engine_domain  LeftPortType=input  RightPortType=generic  SubClassName=solver  Accelerate=off  Profile=off  ResidualTolerance=1e-9  MaxNonlinIter=3  MaxModeIter=2  DoFixedCost=off  UseLocalSampling=off  DoDC=off  LinearAlgebra=Sparse  LocalSolverSampleTime=.001  LocalSolverChoice=NE_BACKWARD_EULER_ADVANCER  UseLocalSolver=off
  Voltage  Measurement : powerlib/Measurements/Voltage Measurement  DialogController=POWERSYS.PowerSysDialog  SystemSampleTime=-1  PhasorSimulation=off  OutputType=Complex  PSBequivalent=0
  Voltage Sensor : fl_lib/Electrical/Electrical Sensors/Voltage Sensor  DialogController=NetworkEngine.DynNeDlgSource  SystemSampleTime=-1  i1_Log=off  v1_Log=off  LocalVarNames=|i1|v1  LocalVarDescs=|i1|v1  LocalVarLogging=[0 0]
  + : PMIOPort  Port=1  Side=Left
  - : PMIOPort  Port=2  Side=Left
  current : Outport
  current1 : Outport  Port=2
  wires:
  PS-Simulink Converter/1 -> Controlled  Current  Source/1
  Current  Measurement/1 -> Scope1/1, Product/2, current/1
  Voltage  Measurement/1 -> Scope1/2, Product/1, current1/1
  Product/1 -> Scope2/1
  connections:
  PV Pannel3/LConn1 -- PV Pannel1/LConn1 -- Current  Sensor/LConn1 -- PV Pannel/LConn1 -- Voltage Sensor/LConn1 -- PV Pannel5/LConn1 -- PV Pannel2/LConn1 -- PV Pannel4/LConn1
  PV Pannel3/LConn2 -- Solver Configuration/RConn1 -- Electrical Reference/LConn1 -- Current  Sensor/RConn2 -- Voltage Sensor/RConn2 -- PV Pannel/LConn2 -- PV Pannel1/LConn2 -- PV Pannel5/LConn2 -- PV Pannel2/LConn2 -- PV Pannel4/LConn2
  Controlled  Current  Source/LConn1 -- Voltage  Measurement/LConn2 -- " R "/RConn1 -- -/RConn1
  Current  Measurement/RConn1 -- Voltage  Measurement/LConn1 -- " R "/LConn1 -- +/RConn1
  Current  Sensor/RConn1 -- PS-Simulink Converter/LConn1
  Current  Measurement/LConn1 -- Controlled  Current  Source/RConn1

== system main1/Subsystem2/LP filter 2nd order ==
  a : Inport  OutDataType=sfix(16)  OutScaling=2^0
  b : Inport  Port=2  OutDataType=sfix(16)  OutScaling=2^0
  c : Inport  Port=3  OutDataType=sfix(16)  OutScaling=2^0
  2nd-Order Filter : powerlib_extras/Control  Blocks/2nd-Order Filter  DialogController=POWERSYS.PowerSysDialog  SystemSampleTime=-1  FilterType=Lowpass  Fo=cutoff_frequency  Zeta=damping_factor  Initialize=off  Vac_Init=[1 45 60]  Vdc_Init=-0.5  PlotResponse=off  param1=[1 500 1]
  2nd-Order Filter1 : powerlib_extras/Control  Blocks/2nd-Order Filter  DialogController=POWERSYS.PowerSysDialog  SystemSampleTime=-1  FilterType=Lowpass  Fo=cutoff_frequency  Zeta=damping_factor  Initialize=off  Vac_Init=[1 45 60]  Vdc_Init=-0.5  PlotResponse=off  param1=[1 500 1]
  2nd-Order Filter2 : powerlib_extras/Control  Blocks/2nd-Order Filter  DialogController=POWERSYS.PowerSysDialog  SystemSampleTime=-1  FilterType=Lowpass  Fo=cutoff_frequency  Zeta=damping_factor  Initialize=off  Vac_Init=[1 45 60]  Vdc_Init=-0.5  PlotResponse=off  param1=[1 500 1]
  A : Outport  OutDataType=sfix(16)  OutScaling=2^0
  B : Outport  Port=2  OutDataType=sfix(16)  OutScaling=2^0
  C : Outport  Port=3  OutDataType=sfix(16)  OutScaling=2^0
  wires:
  a/1 -> 2nd-Order Filter/1
  2nd-Order Filter/1 -> A/1
  b/1 -> 2nd-Order Filter1/1
  2nd-Order Filter1/1 -> B/1
  c/1 -> 2nd-Order Filter2/1
  2nd-Order Filter2/1 -> C/1

== system main1/Subsystem2/Subsystem1 ==
  ref_frequency : Inport
  direction : Inport  Port=2
  carrier_frequency : Inport  Port=3
  duty_ratio : Inport  Port=4
  Angle_generator : Subsystem
  Demux : Demux  Outputs=6
  Logical Operator : Logic  AllPortsSameDT=off  OutDataTypeMode=boolean  LogicDataType=fixdt(0, 8)  OutDataTypeStr=boolean
  PQ : Subsystem
  VF : Subsystem
  s1 : Outport
  s2 : Outport  Port=2
  s3 : Outport  Port=3
  s4 : Outport  Port=4
  s5 : Outport  Port=5
  s6 : Outport  Port=6
  wires:
  Angle_generator/1(ramp_out) -> VF/1(ramp_inp)
  Demux/1 -> s1/1
  ref_frequency/1 -> Angle_generator/1(freq_inp)
  Demux/2 -> s2/1
  Demux/3 -> s3/1
  Demux/4 -> s4/1
  Demux/5 -> s5/1
  direction/1 -> VF/2(dir)
  Demux/6 -> s6/1
  carrier_frequency/1 -> PQ/1(carrier_frequency)
  duty_ratio/1 -> PQ/2(%duty_ratio)
  VF/1(gate_logic) -> Logical Operator/1
  PQ/1(PWM_signal) -> Logical Operator/2
  Logical Operator/1 -> Demux/1

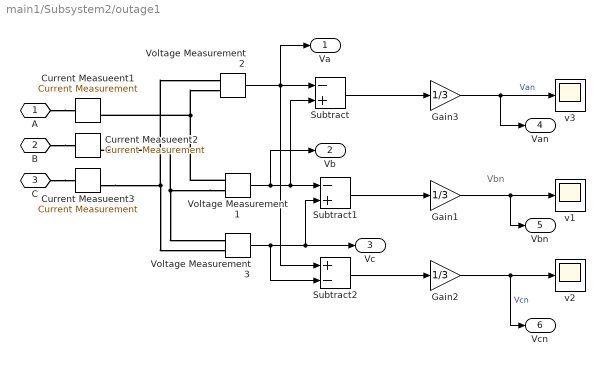
== system main1/Subsystem2/outage1 ==
  note: Vbn
  Current Measueent1 : powerlib/Measurements/Current Measurement  DialogController=POWERSYS.PowerSysDialog  SystemSampleTime=-1  PhasorSimulation=off  OutputType=Complex  PSBequivalent=0
  Current Measueent2 : powerlib/Measurements/Current Measurement  DialogController=POWERSYS.PowerSysDialog  SystemSampleTime=-1  PhasorSimulation=off  OutputType=Complex  PSBequivalent=0
  Current Measueent3 : powerlib/Measurements/Current Measurement  DialogController=POWERSYS.PowerSysDialog  SystemSampleTime=-1  PhasorSimulation=off  OutputType=Complex  PSBequivalent=0
  Gain1 : Gain  Gain=1/3  ParameterDataType=sfix(16)  ParameterScaling=2^0  OutDataType=sfix(16)  OutScaling=2^0
  Gain2 : Gain  Gain=1/3  ParameterDataType=sfix(16)  ParameterScaling=2^0  OutDataType=sfix(16)  OutScaling=2^0
  Gain3 : Gain  Gain=1/3  ParameterDataType=sfix(16)  ParameterScaling=2^0  OutDataType=sfix(16)  OutScaling=2^0
  Subtract : Sum  Inputs=-+  OutDataType=sfix(16)  OutScaling=2^-10
  Subtract1 : Sum  Inputs=-+  OutDataType=sfix(16)  OutScaling=2^-10
  Subtract2 : Sum  Inputs=+-  OutDataType=sfix(16)  OutScaling=2^-10
  Voltage Measurement1 : powerlib/Measurements/Voltage Measurement  DialogController=POWERSYS.PowerSysDialog  SystemSampleTime=-1  PhasorSimulation=off  OutputType=Complex  PSBequivalent=0
  Voltage Measurement2 : powerlib/Measurements/Voltage Measurement  DialogController=POWERSYS.PowerSysDialog  SystemSampleTime=-1  PhasorSimulation=off  OutputType=Complex  PSBequivalent=0
  Voltage Measurement3 : powerlib/Measurements/Voltage Measurement  DialogController=POWERSYS.PowerSysDialog  SystemSampleTime=-1  PhasorSimulation=off  OutputType=Complex  PSBequivalent=0
  v1 : Scope
      settings: SaveName=ScopeData25  MaxDataPoints=5000000
  v2 : Scope
      settings: SaveName=ScopeData26  MaxDataPoints=5000000
  v3 : Scope
      settings: YMin=-300  YMax=300  SaveName=ScopeData27  MaxDataPoints=5000000
  A : PMIOPort  Port=1  Side=Left
  B : PMIOPort  Port=2  Side=Left
  C : PMIOPort  Port=3  Side=Left
  Va : Outport  OutDataType=sfix(16)  OutScaling=2^0
  Vb : Outport  Port=2  OutDataType=sfix(16)  OutScaling=2^0
  Vc : Outport  Port=3  OutDataType=sfix(16)  OutScaling=2^0
  Van : Outport  Port=4  OutDataType=sfix(16)  OutScaling=2^0
  Vbn : Outport  Port=5  OutDataType=sfix(16)  OutScaling=2^0
  Vcn : Outport  Port=6  OutDataType=sfix(16)  OutScaling=2^0
  wires:
  Gain2/1 -> v2/1, Vcn/1  "Vcn"
  Subtract2/1 -> Gain2/1
  Gain1/1 -> v1/1, Vbn/1
  Subtract1/1 -> Gain1/1
  Voltage Measurement3/1 -> Subtract2/2, Subtract1/2, Vc/1
  Gain3/1 -> v3/1, Van/1  "Van"
  Subtract/1 -> Gain3/1
  Voltage Measurement1/1 -> Subtract/2, Subtract1/1, Vb/1
  Voltage Measurement2/1 -> Subtract/1, Subtract2/1, Va/1
  connections:
  Voltage Measurement1/LConn1 -- Current Measueent1/RConn1 -- Voltage Measurement2/LConn2
  Voltage Measurement1/LConn2 -- Current Measueent2/RConn1 -- Voltage Measurement3/LConn1
  Current Measueent3/RConn1 -- Voltage Measurement2/LConn1 -- Voltage Measurement3/LConn2
  A/RConn1 -- Current Measueent1/LConn1
  B/RConn1 -- Current Measueent2/LConn1
  C/RConn1 -- Current Measueent3/LConn1
